simulink model "HCS_model"  (R2022b)
settings: Solver=VariableStepAuto  StartTime=0.0  StopTime=t_sample*n_sample  MaxStep=5  MinStep=1  RelTol=1e-3
values from neighbouring files (symbols this model uses):
  air_den = 1.225    [wind_turbine_parameters.m]
  l1 = 56    [wind_turbine_parameters.m]
  t_sample = 10*60    (= 600)    [wind_turbine_parameters.m]
undefined symbols (not defined in the file or in its folder): pitch_deg
libraries: simulink x1, spsWindTurbineLib x1
settings Model: Creator=luan  LastModifiedBy=marina
settings SolverCC: ZeroCrossAlgorithm=Adaptive
settings DebuggingCC: IgnoredZcDiagnostic=none

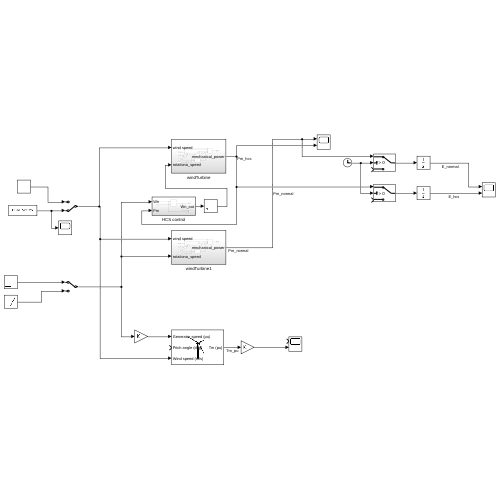
[thumbnail: Simulink's stored preview of the top-level diagram]
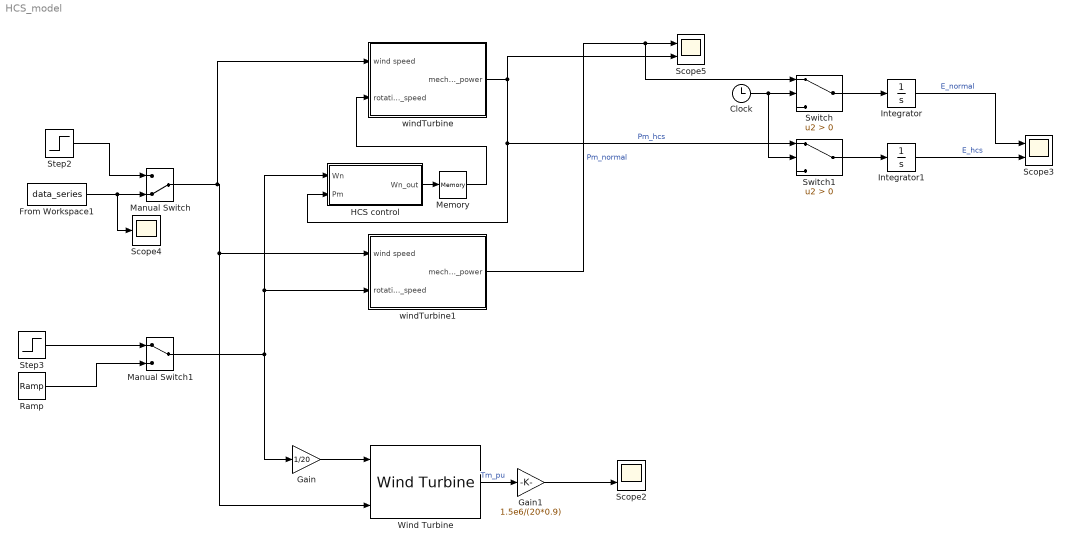
== system HCS_model ==
  Clock : Clock
  From Workspace1 : FromWorkspace  VariableName=data_series  SampleTime=t_sample  OutputAfterFinalValue=Setting to zero
  Gain : Gain  Gain=1/20
  Gain1 : Gain  Gain=1.5e6/(20*0.9)
  HCS control : Subsystem
  Integrator : Integrator
  Integrator1 : Integrator
  Manual Switch : ManualSwitch  CurrentSetting=0
  Manual Switch1 : ManualSwitch
  Memory : Memory
  Ramp : simulink/Sources/Ramp  slope=0.000007  start=0  InitialOutput=0.0001
  Scope2 : Scope  NumInputPorts=2
  Scope3 : Scope  NumInputPorts=2
  Scope4 : Scope
  Scope5 : Scope  NumInputPorts=2
  Step2 : Step  Time=0  After=11  SampleTime=0
  Step3 : Step  Time=0  SampleTime=0
  Switch : Switch  Criteria=u2 > Threshold  SaturateOnIntegerOverflow=off  InputSameDT=off
  Switch1 : Switch  Criteria=u2 > Threshold  SaturateOnIntegerOverflow=off  InputSameDT=off
  Wind Turbine : spsWindTurbineLib/Wind Turbine  Pnom=1.5e6  Pelec_base=1.5e6/0.9  wind_base=20  P_wind_base=0.73  speed_nom=1.2  pitch_angle=0  c1_c6="[0.51763          116          0.4            5           21     0.006795]"  cp_nom=0.48  lambda_nom=8.1
  windTurbine : Subsystem
  windTurbine1 : Subsystem
  wires:
  Gain/1 -> Wind Turbine/1
  Wind Turbine/1 -> Gain1/1  "Tm_pu"
  Gain1/1 -> Scope2/2
  windTurbine1/1(mechanical_power) -> Switch/1, Scope5/1  "Pm_normal"
  windTurbine/1(mechanical_power) -> Scope5/2, Switch1/1, HCS control/2(Pm)  "Pm_hcs"
  Step2/1 -> Manual Switch/1
  Manual Switch/1 -> windTurbine/1(wind speed), Wind Turbine/3, windTurbine1/1(wind speed)
  From Workspace1/1 -> Scope4/1, Manual Switch/2
  Step3/1 -> Manual Switch1/1
  Ramp/1 -> Manual Switch1/2
  Manual Switch1/1 -> windTurbine1/2(rotationa_speed), HCS control/1(Wn), Gain/1
  HCS control/1(Wn_out) -> Memory/1
  Memory/1 -> windTurbine/2(rotationa_speed)
  Integrator/1 -> Scope3/1  "E_normal"
  Integrator1/1 -> Scope3/2  "E_hcs"
  Clock/1 -> Switch1/2, Switch/2
  Switch/1 -> Integrator/1
  Switch1/1 -> Integrator1/1

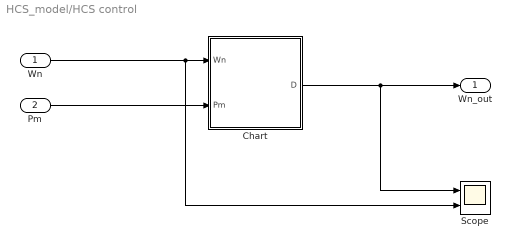
== system HCS_model/HCS control ==
  Wn : Inport
  Pm : Inport  Port=2
  Chart : Stateflow chart  TreatAsAtomicUnit=on
  Scope : Scope  NumInputPorts=2
  Wn_out : Outport
  wires:
  Pm/1 -> Chart/2(Pm)
  Wn/1 -> Scope/2, Chart/1(Wn)
  Chart/1(D) -> Scope/1, Wn_out/1

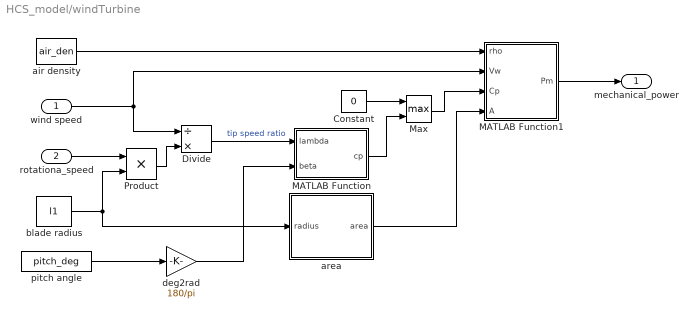
== system HCS_model/windTurbine ==
  wind speed : Inport
  rotationa_speed : Inport  Port=2
  Constant : Constant  Value=0
  Divide : Product  Inputs=/*
  MATLAB Function : MATLAB Function  TreatAsAtomicUnit=on
  MATLAB Function1 : MATLAB Function  TreatAsAtomicUnit=on
  Max : MinMax  Function=max  Inputs=2
  Product : Product
  air density : Constant  Value=air_den
  area : Subsystem
  blade radius : Constant  Value=l1
  deg2rad : Gain  Gain=180/pi
  pitch angle : Constant  Value=pitch_deg
  mechanical_power : Outport
  wires:
  Product/1 -> Divide/2
  wind speed/1 -> Divide/1, MATLAB Function1/2(Vw)
  Divide/1 -> MATLAB Function/1(lambda)  "tip speed ratio"
  MATLAB Function1/1(Pm) -> mechanical_power/1
  rotationa_speed/1 -> Product/1
  air density/1 -> MATLAB Function1/1(rho)
  area/1(area) -> MATLAB Function1/4(A)
  blade radius/1 -> Product/2, area/1(radius)
  deg2rad/1 -> MATLAB Function/2(beta)
  Max/1 -> MATLAB Function1/3(Cp)
  MATLAB Function/1(cp) -> Max/2
  Constant/1 -> Max/1
  pitch angle/1 -> deg2rad/1

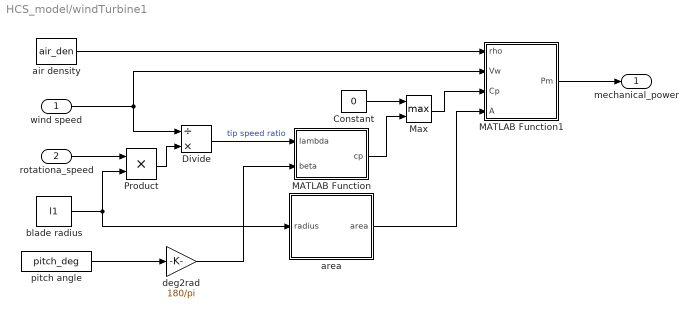
== system HCS_model/windTurbine1 ==
  wind speed : Inport
  rotationa_speed : Inport  Port=2
  Constant : Constant  Value=0
  Divide : Product  Inputs=/*
  MATLAB Function : MATLAB Function  TreatAsAtomicUnit=on
  MATLAB Function1 : MATLAB Function  TreatAsAtomicUnit=on
  Max : MinMax  Function=max  Inputs=2
  Product : Product
  air density : Constant  Value=air_den
  area : Subsystem
  blade radius : Constant  Value=l1
  deg2rad : Gain  Gain=180/pi
  pitch angle : Constant  Value=pitch_deg
  mechanical_power : Outport
  wires:
  Product/1 -> Divide/2
  wind speed/1 -> Divide/1, MATLAB Function1/2(Vw)
  Divide/1 -> MATLAB Function/1(lambda)  "tip speed ratio"
  MATLAB Function1/1(Pm) -> mechanical_power/1
  rotationa_speed/1 -> Product/1
  air density/1 -> MATLAB Function1/1(rho)
  area/1(area) -> MATLAB Function1/4(A)
  blade radius/1 -> Product/2, area/1(radius)
  deg2rad/1 -> MATLAB Function/2(beta)
  Max/1 -> MATLAB Function1/3(Cp)
  MATLAB Function/1(cp) -> Max/2
  Constant/1 -> Max/1
  pitch angle/1 -> deg2rad/1

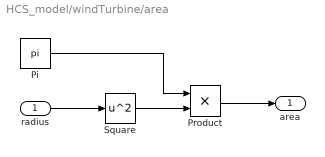
== system HCS_model/windTurbine/area ==
  radius : Inport
  Pi : Constant  Value=pi  OutDataTypeStr=Inherit: Inherit via back propagation
  Product : Product
  Square : Math  Operator=square
  area : Outport
  wires:
  radius/1 -> Square/1
  Square/1 -> Product/2
  Pi/1 -> Product/1
  Product/1 -> area/1

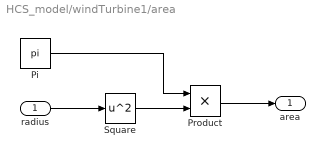
== system HCS_model/windTurbine1/area ==
  radius : Inport
  Pi : Constant  Value=pi  OutDataTypeStr=Inherit: Inherit via back propagation
  Product : Product
  Square : Math  Operator=square
  area : Outport
  wires:
  radius/1 -> Square/1
  Square/1 -> Product/2
  Pi/1 -> Product/1
  Product/1 -> area/1

== stateflow chart HCS_model/HCS control/Chart ==
  state stationary
    entry:
    D = Wn;
  state init_
    entry:
    D = Wn;
    pt_1 = 0;
    d_ = d;
  state measure
    entry:
    dp = Pm - pt_1;
    pt_1 = Pm;
  state decrease
    entry:
    d_ = - d_;
  state increase
    entry:
    d_ = d_;
  state perturb_
    entry:
    D = D + d_;
  measure -> stationary [order 3] : [abs(dp)< 500]
  stationary -> measure : [after(delay,sec)]
  (default) -> init_
  measure -> decrease [order 2] : [dp < 0]
  init_ -> measure
  perturb_ -> measure : [after(delay,sec)]
  decrease -> perturb_
  measure -> increase [order 1] : [dp > 0]
  increase -> perturb_
  data: Wn input; Pm input; D output; delay constant double =5; d constant double =0.05; pt_1 local; dp local; d_ local

== matlab function HCS_model/windTurbine/MATLAB Function ==
  data: lambda input; cp output; beta input
function cp = fcn(lambda, beta)

k = load('coefficients.mat');
lambda_i =  1/(1/(lambda + 0.08*beta) - 0.035/(1+beta*beta*beta));

% Debug
% lambda_i
% k.k1 *(k.k2/lambda_i - k.k3*beta - k.k4*power(beta, k.k5) -k.k6)*exp(-k.k7/lambda_i)

cp = k.k1 *(k.k2/lambda_i - k.k3*beta - k.k4*power(beta, k.k5) -k.k6)*exp(-k.k7/lambda_i);

== matlab function HCS_model/windTurbine1/MATLAB Function ==
  data: lambda input; cp output; beta input
function cp = fcn(lambda, beta)

k = load('coefficients.mat');
lambda_i =  1/(1/(lambda + 0.08*beta) - 0.035/(1+beta*beta*beta));

% Debug
% lambda_i
% k.k1 *(k.k2/lambda_i - k.k3*beta - k.k4*power(beta, k.k5) -k.k6)*exp(-k.k7/lambda_i)

cp = k.k1 *(k.k2/lambda_i - k.k3*beta - k.k4*power(beta, k.k5) -k.k6)*exp(-k.k7/lambda_i);

== matlab function HCS_model/windTurbine1/MATLAB Function1 ==
  data: rho input; Vw input; Pm output; Cp input; A input
function Pm = fcn(rho, Vw, Cp, A)

Pm = 0.5* Cp* rho* A* power(Vw, 3);

== matlab function HCS_model/windTurbine/MATLAB Function1 ==
  data: rho input; Vw input; Pm output; Cp input; A input
function Pm = fcn(rho, Vw, Cp, A)

Pm = 0.5* Cp* rho* A* power(Vw, 3);
